simulink subsystem "halfCosineRamp"  (R2024b)
settings: Solver=VariableStepAuto  StartTime=0.0  StopTime=10.0  RelTol=1e-3
settings Model: Creator=phippold  LastModifiedBy=phippold

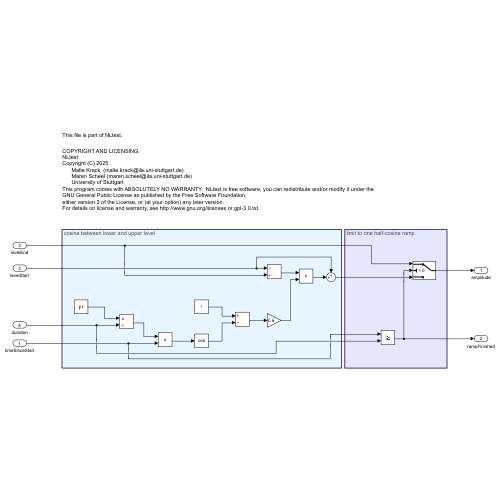
[thumbnail: Simulink's stored preview of the top-level diagram]
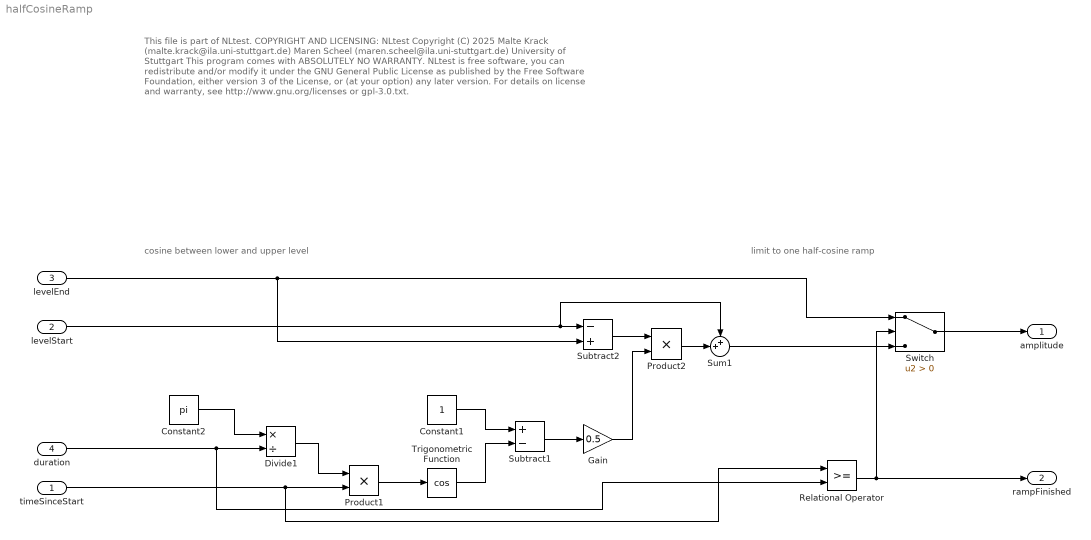
== system halfCosineRamp ==
  note: limit to one half-cosine ramp
  note: cosine between lower and upper level
  note: This file is part of NLtest.
      |
      | COPYRIGHT AND LICENSING:
      | NLtest
      | Copyright (C) 2025
      | Malte Krack (malte.krack@ila.uni-stuttgart.de)
      | Maren Scheel (maren.scheel@ila.uni-stuttgart.de)
      | University of Stuttgart
      | This program comes with ABSOLUTELY NO WARRANTY. NLtest is free software, you can redistribute and/or modify it under the GNU General Public License as published by the Free Software Foundation,
      | either version 3 of the License, or (at your option) any later version.
      | For details on license and warranty, see http://www.gnu.org/licenses or gpl-3.0.txt.
  timeSinceStart : Inport
  levelStart : Inport  Port=2
  "levelEnd " : Inport  Port=3
  duration : Inport  Port=4
  Constant1 : Constant
  Constant2 : Constant  Value=pi
  Divide1 : Product  Inputs=*/
  Gain : Gain  Gain=0.5
  Product1 : Product
  Product2 : Product
  Relational Operator : RelationalOperator  OutDataTypeStr=boolean  RndMeth=Simplest  InputSameDT=off
  Subtract1 : Sum  Inputs=+-
  Subtract2 : Sum  Inputs=-+
  Sum1 : Sum  Inputs=++|
  Switch : Switch  Criteria=u2 > Threshold  SaturateOnIntegerOverflow=off  InputSameDT=off
  Trigonometric Function : Trigonometry  Operator=cos
  amplitude : Outport
  rampFinished : Outport  Port=2
  wires:
  duration/1 -> Divide1/2, Relational Operator/2
  Relational Operator/1 -> Switch/2, rampFinished/1
  timeSinceStart/1 -> Product1/2, Relational Operator/1
  "levelEnd "/1 -> Subtract2/2, Switch/1
  Switch/1 -> amplitude/1
  Product2/1 -> Sum1/2
  Subtract2/1 -> Product2/1
  levelStart/1 -> Subtract2/1, Sum1/1
  Constant2/1 -> Divide1/1
  Divide1/1 -> Product1/1
  Product1/1 -> Trigonometric Function/1
  Trigonometric Function/1 -> Subtract1/2
  Constant1/1 -> Subtract1/1
  Subtract1/1 -> Gain/1
  Gain/1 -> Product2/2
  Sum1/1 -> Switch/3
